simulink model "w1954016_simulink"  (R2023b)
settings: Solver=VariableStepAuto  StartTime=0.0  StopTime=10  RelTol=1e-3
settings Model: Creator=chama  LastModifiedBy=chama

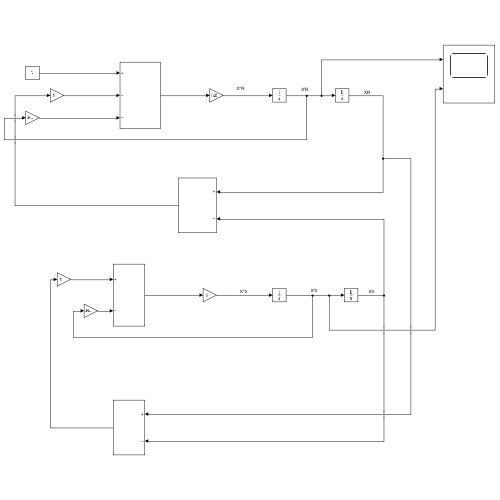
[thumbnail: Simulink's stored preview of the top-level diagram]
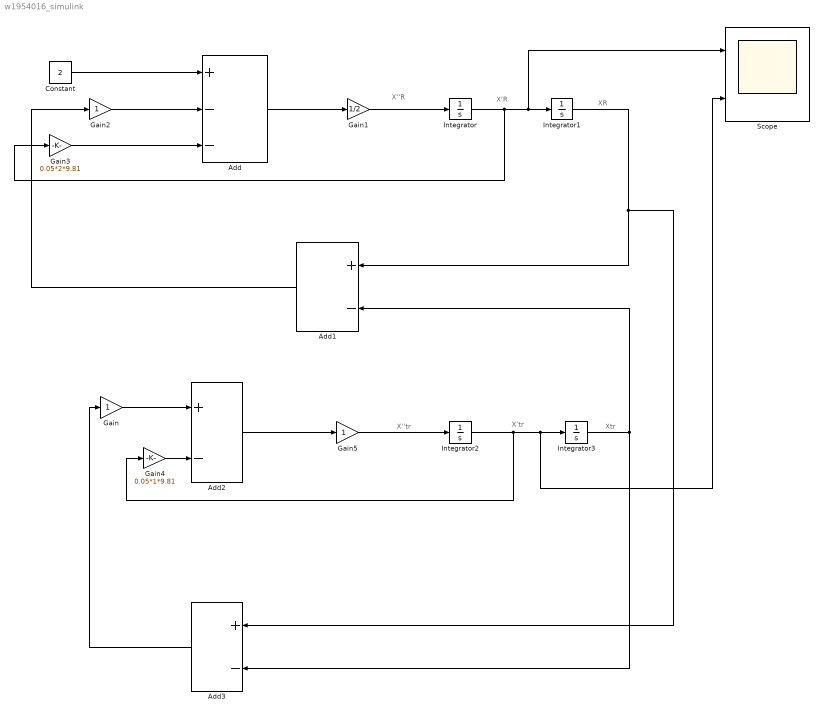
== system w1954016_simulink ==
  note: Xtr
  note: XR
  note: X'tr
  note: X''tr
  note: X'R
  note: X''R
  Add : Sum  Inputs=+--
  Add1 : Sum  Inputs=+-
  Add2 : Sum  Inputs=+-
  Add3 : Sum  Inputs=+-
  Constant : Constant  Value=2
  Gain : Gain
  Gain1 : Gain  Gain=1/2
  Gain2 : Gain
  Gain3 : Gain  Gain=0.05*2*9.81
  Gain4 : Gain  Gain=0.05*1*9.81
  Gain5 : Gain
  Integrator{,1..3} (4 alike) : Integrator
  Scope : Scope  NumInputPorts=2
  wires:
  Constant/1 -> Add/1
  Gain2/1 -> Add/2
  Gain3/1 -> Add/3
  Add1/1 -> Gain2/1
  Add/1 -> Gain1/1
  Gain1/1 -> Integrator/1
  Integrator/1 -> Scope/1, Integrator1/1, Gain3/1
  Integrator1/1 -> Add1/1, Add3/1
  Gain/1 -> Add2/1
  Add3/1 -> Gain/1
  Gain4/1 -> Add2/2
  Add2/1 -> Gain5/1
  Gain5/1 -> Integrator2/1
  Integrator3/1 -> Add1/2, Add3/2
  Integrator2/1 -> Gain4/1, Scope/2, Integrator3/1
